simulink model "Modelo_segundo_orden_sist_no_lineal_obt_datos"  (R2016a)
settings: Solver=VariableStepAuto  StartTime=0.0  StopTime=300  RelTol=1e-3
settings Model: Creator=Daniel  LastModifiedBy=Daniel

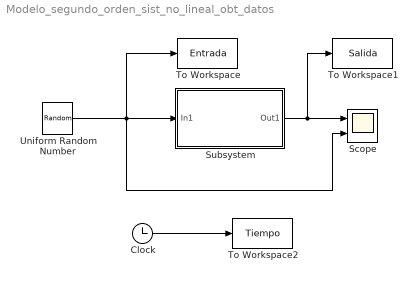
== system Modelo_segundo_orden_sist_no_lineal_obt_datos ==
  Clock : Clock
  Scope : Scope  NumInputPorts=2
  Subsystem : Subsystem
  To Workspace : ToWorkspace  VariableName=Entrada  SampleTime=0.2
  To Workspace1 : ToWorkspace  VariableName=Salida  SampleTime=0.2
  To Workspace2 : ToWorkspace  VariableName=Tiempo  SampleTime=0.2
  Uniform Random Number : UniformRandomNumber  Minimum=0  Maximum=10  SampleTime=10
  wires:
  Uniform Random Number/1 -> To Workspace/1, Subsystem/1(In1), Scope/2
  Clock/1 -> To Workspace2/1
  Subsystem/1(Out1) -> Scope/1, To Workspace1/1

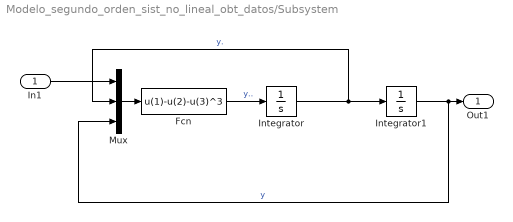
== system Modelo_segundo_orden_sist_no_lineal_obt_datos/Subsystem ==
  In1 : Inport
  Fcn : Fcn  Expr=u(1)-u(2)-u(3)^3
  Integrator : Integrator
  Integrator1 : Integrator
  Mux : Mux  Inputs=3
  Out1 : Outport
  wires:
  In1/1 -> Mux/1
  Mux/1 -> Fcn/1
  Fcn/1 -> Integrator/1  "y.."
  Integrator/1 -> Mux/2, Integrator1/1  "y."
  Integrator1/1 -> Mux/3, Out1/1  "y"
